simulink model "Fruit"  (Simulink 7.7)
settings: Solver=FixedStepDiscrete  StartTime=0.0  StopTime=inf  RelTol=1e-3
libraries: vipsnks x3, nid_lib x2
settings Model: Creator=Hayyaan  LastModifiedBy=Hayyaan
settings SolverCC: AutoInsertRateTranBlk=on
settings DataIOCC: SaveOutput=off  SaveTime=off
settings OptimizationCC: InlineParams=on  InlineInvariantSignals=on  StateBitsets=on  DataBitsets=on  UseTempVars=on  ZeroExternalMemoryAtStartup=off  ZeroInternalMemoryAtStartup=off  NoFixptDivByZeroProtection=on  OptimizeModelRefInitCode=on  LifeSpan=1
settings HardwareCC: ProdIntDivRoundTo=Floor  ProdEndianess=LittleEndian  ProdHWDeviceType=Generic->Custom
settings RTWCC: SystemTargetFile=ert.tlc  TLCOptions=-p0  GenCodeOnly=on  TemplateMakefile=ert_default_tmf  Description=Embedded Coder  GenerateReport=on  RTWVerbose=off  ProcessScript=ert_make_rtw_hook  IncludeHyperlinkInReport=on  LaunchReport=on
settings CodeAppCC: ForceParamTrailComments=on  IgnoreCustomStorageClasses=off  SimulinkDataObjDesc=on  CustomSymbolStrGlobalVar=rt$N$M  CustomSymbolStrType=$N$M  CustomSymbolStrFcn=$N$M$F  CustomSymbolStrMacro=$N$M  InsertBlockDesc=on
settings ERTTargetCC: TargetFunctionLibrary=ISO_C  FunctionExecutionProfile=off  MultiwordLength=2048  GenerateSampleERTMain=on  IncludeMdlTerminateFcn=off  SuppressErrorStatus=on  SupportAbsoluteTime=off  SupportNonFinite=off  SupportComplex=off  PurelyIntegerCode=on  InlinedParameterPlacement=NonHierarchical  RootIOFormat=Structure reference  ERTCustomFileTemplate=example_file_process.tlc  ConvertIfToSwitch=off

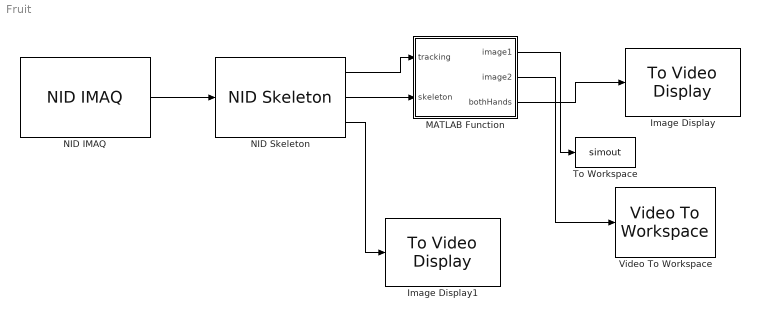
== system Fruit ==
  Image Display : vipsnks/To Video Display  inputType=Obsolete  imagePorts=One multidimensional signal  OutputDevice=On-screen video monitor  fullScreen=off  videoWindowX=345  videoWindowY=442  saveWindowSize=off  videoWindowWidth=640  videoWindowHeight=480  dataOrg=Column-major  openAtMdlStart=on  isWindowOpen=off  inputColorFormat=RGB
  Image Display1 : vipsnks/To Video Display  inputType=Obsolete  imagePorts=One multidimensional signal  OutputDevice=On-screen video monitor  fullScreen=off  videoWindowX=1210  videoWindowY=406  saveWindowSize=off  videoWindowWidth=640  videoWindowHeight=480  dataOrg=Column-major  openAtMdlStart=on  isWindowOpen=off  inputColorFormat=RGB
  MATLAB Function : Stateflow chart  TreatAsAtomicUnit=on
  NID IMAQ : nid_lib/NID IMAQ  imaq_depth=off  imaq_motion=off  imaq_image=off  view_point=on  imaq_skeleton=on  imaq_ir=off  mirror_image=on  imaq_sample_time=1/30  res_fps=VGA (640x480): 30 FPS  angle=-20  near_mode=off
  NID Skeleton : nid_lib/NID Skeleton  conv_XYZ_RW=off  viewer=on  needPsiPose=off
  To Workspace : ToWorkspace  VariableName=simout  SampleTime=-1  SaveFormat=Structure
  Video To Workspace : vipsnks/Video To Workspace  VariableName=vout  NumInputs=1  DataLimit=10  DecimationFactor=1  LogFi=off  InPortLabels=R|G|B
  wires:
  NID IMAQ/1 -> NID Skeleton/1
  NID Skeleton/1 -> MATLAB Function/1(tracking)
  NID Skeleton/2 -> MATLAB Function/2(skeleton)
  MATLAB Function/3(bothHands) -> Image Display/1
  NID Skeleton/3 -> Image Display1/1
  MATLAB Function/1(image1) -> To Workspace/1
  MATLAB Function/2(image2) -> Video To Workspace/1

== matlab function MATLAB Function ==
  data: tracking input double; image1 output double; skeleton input double; image2 output double; bothHands output double
function [image1,image2,bothHands] = fcn(tracking,skeleton)
%#codegen
if tracking ==1
    image1 = logical(zeros(480,640));
    imageCoordinates=zeros(2,15);
    imageCoordinates(1,:)=skeleton(:,:,1)*1000;
    imageCoordinates(2,:)=skeleton(:,:,2)*1000;
    p.rhand = GetJointCoordinates('SKELETON_RIGHT_HAND',imageCoordinates);
    p.lhand = GetJointCoordinates('SKELETON_LEFT_HAND',imageCoordinates);
    [X,Y] = meshgrid(1:640,1:480);
    
    image1 = (((X-p.rhand(1)).^2 + (Y-p.rhand(2)).^2 <20^2) == 1);
    image2 = (((X-p.lhand(1)).^2 + (Y-p.lhand(2)).^2 <20^2) == 1);
    bothHands = image2 | image1;
else
    image1 = logical(zeros(480,640));
    image2 = logical(zeros(480,640));
    bothHands = logical(zeros(480,640));
end
